simulink model "sistema_mecanico"  (R2016b)
settings: Solver=VariableStepAuto  StartTime=0.0  StopTime=10.0  RelTol=1e-3
values from neighbouring files (symbols this model uses):
  Beq = bm+(bl)/r^2    (= 1.5e-05)    [c4ModeloCompleto_var.m]
  Jeq = Jm+(Jl/r^2)    (= 5.65099476805e-06)    [c4ModeloCompleto_var.m]
  r = 314.3008    [c4ModeloCompleto.m]    (also in c4ModeloCompleto_var.m)
settings Model: Creator=agustin  LastModifiedBy=agustin

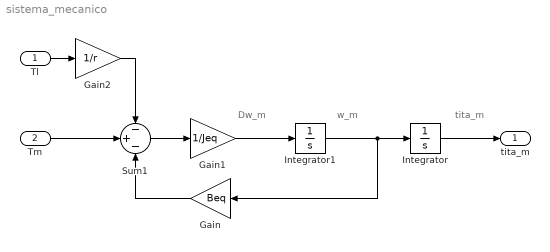
== system sistema_mecanico ==
  note: tita_m
  note: w_m
  note: Dw_m
  Tl : Inport
  Tm : Inport  Port=2
  Gain : Gain  Gain=Beq
  Gain1 : Gain  Gain=1/Jeq
  Gain2 : Gain  Gain=1/r
  Integrator : Integrator
  Integrator1 : Integrator
  Sum1 : Sum  Inputs=-+-
  tita_m : Outport
  wires:
  Gain1/1 -> Integrator1/1
  Integrator1/1 -> Integrator/1, Gain/1
  Gain/1 -> Sum1/3
  Tl/1 -> Gain2/1
  Sum1/1 -> Gain1/1
  Integrator/1 -> tita_m/1
  Tm/1 -> Sum1/2
  Gain2/1 -> Sum1/1
